simulink model "EnableBio1"  (R2017b)
settings: Solver=FixedStepDiscrete  StartTime=0.0  StopTime=10.0  FixedStep=0.200000  RelTol=1e-3  EnableMultiTasking=on
PreLoadFcn:
  | cellInfo = {
  |     { ...
  |          'cmp_cmd_msg' , ...
  |          '', ...
  |          sprintf(''), {  ...
  |                {  'apid', 1, 'uint16', -1, 'real', 'Sample' }; ...
  |                {  'sequence', 1, 'uint16', -1, 'real', 'Sample' }; ...
  |                {  'length', 1, 'uint16', -1, 'real', 'Sample' }; ...
  |                {  'command_id', 1, 'uint8', -1, 'real', 'Sample' }; ...
  |                {  'checksum', 1, 'uint8', -1, 'real', 'Sample' }; ...
  |                {  'params', 34, 'uint8', -1, 'real', 'Sample' }; ...
  |          }
  |     }
  | };
  | Simulink.Bus.cellToObject(cellInfo);
undefined symbols (not defined in the file): command_id, params, sequence
settings Model: Creator=hbourbou  LastModifiedBy=hbourbou
settings DataIOCC: LimitDataPoints=on
settings OptimizationCC: LifeSpan=inf
settings DebuggingCC: SFUnexpectedBacktrackingDiag=warning  SFNoUnconditionalDefaultTransitionDiag=warning  SFExecutionAtInitializationDiag=none
settings HardwareCC: ProdBitPerSizeT=32  ProdBitPerPtrDiffT=32  ProdWordSize=32  ProdHWDeviceType=Specified
settings ModelReferenceCC: PropagateSignalLabelsOutOfModel=off
settings CodeAppCC: StateflowObjectComments=on
settings GRTTargetCC: TargetLangStandard=C89/C90 (ANSI)
settings ConfigComp: CovMetricSettings=dw  CovHtmlReporting=on  CovSaveCumulativeToWorkspaceVar=on  CovSaveSingleToWorkspaceVar=on  CovExternalEMLEnable=off

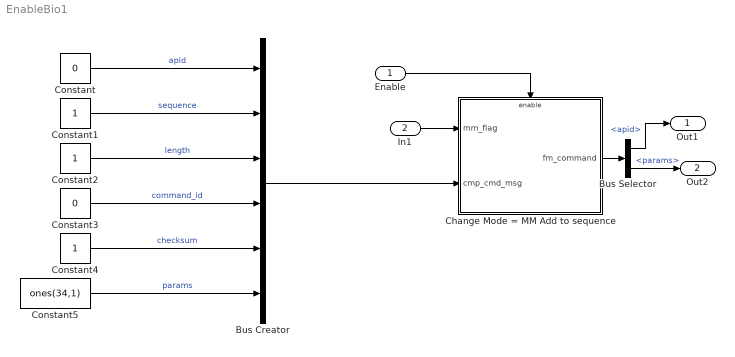
== system EnableBio1 ==
  Enable : Inport  OutDataTypeStr=boolean
  In1 : Inport  Port=2  OutDataTypeStr=uint8
  Bus Creator : BusCreator  Inputs=6  OutDataTypeStr=Bus: cmp_cmd_msg  NonVirtualBus=on
      settings: InheritFromInputs=off
  Bus Selector : BusSelector  OutputSignals=apid,params
  Change Mode = MM Add to sequence : Subsystem  TreatAsAtomicUnit=on
      settings: MinAlgLoopOccurrences=on
  Constant : Constant  Value=0  OutDataTypeStr=uint16
  Constant1 : Constant  OutDataTypeStr=uint16
  Constant2 : Constant  OutDataTypeStr=uint16
  Constant3 : Constant  Value=0  OutDataTypeStr=uint8
  Constant4 : Constant  OutDataTypeStr=uint8
  Constant5 : Constant  Value=ones(34,1)  OutDataTypeStr=uint8
  Out1 : Outport
  Out2 : Outport  Port=2
  wires:
  Change Mode = MM Add to sequence/1(fm_command) -> Bus Selector/1
  Enable/1 -> Change Mode = MM Add to sequence/Enable
  In1/1 -> Change Mode = MM Add to sequence/1(mm_flag)
  Constant4/1 -> Bus Creator/5  "checksum"
  Constant/1 -> Bus Creator/1  "apid"
  Constant5/1 -> Bus Creator/6  "params"
  Bus Creator/1 -> Change Mode = MM Add to sequence/2(cmp_cmd_msg)
  Constant1/1 -> Bus Creator/2  "sequence"
  Constant3/1 -> Bus Creator/4  "command_id"
  Constant2/1 -> Bus Creator/3  "length"
  Bus Selector/1 -> Out1/1  "<apid>"
  Bus Selector/2 -> Out2/1  "<params>"

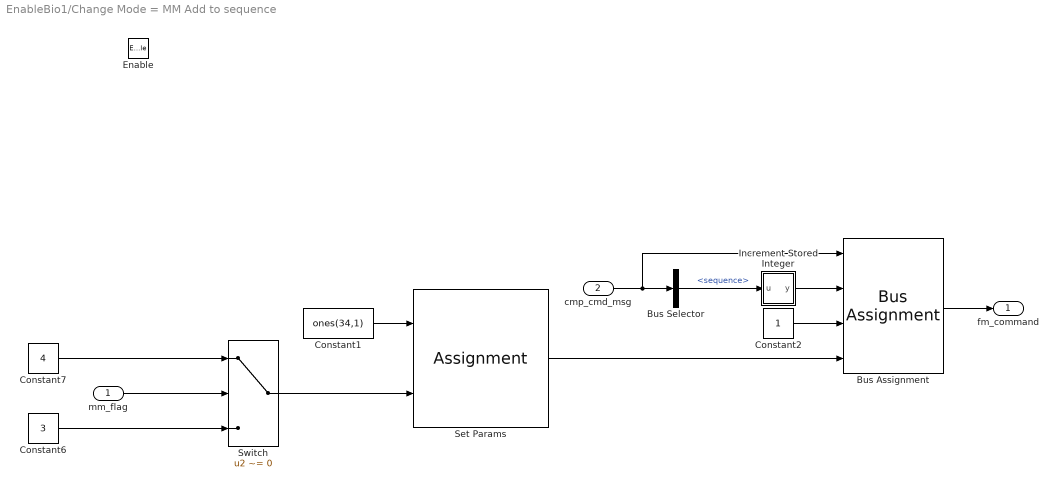
== system EnableBio1/Change Mode = MM Add to sequence ==
  mm_flag : Inport  OutDataTypeStr=uint8
  cmp_cmd_msg : Inport  Port=2  OutDataTypeStr=Bus: cmp_cmd_msg
  Enable : EnablePort
  Bus Assignment : BusAssignment  AssignedSignals=sequence,command_id,params
  Bus Selector : BusSelector  OutputSignals=sequence
  Constant1 : Constant  Value=ones(34,1)  OutDataTypeStr=uint8
  Constant2 : Constant  OutDataTypeStr=uint8
  Constant6 : Constant  Value=3  OutDataTypeStr=uint8
  Constant7 : Constant  Value=4  OutDataTypeStr=uint8
  Increment Stored Integer : Subsystem  AncestorBlock=|  TreatAsAtomicUnit=on  mask(Stored Integer Value Increment){}
      | simulink/Additional Math
      | & Discrete/Additional Math:
      | Increment - Decrement/Increment
      | Stored Integer
      mask help: Simulink:masks:StoredIntegerValueIncrement_MD
      settings: MinAlgLoopOccurrences=on
      mask Display: disp('Q++')
  Set Params : Assignment  DiagnosticForDimensions=Warning  IndexOptions=Index vector (dialog)  Indices=1  OutputSizes=1
  Switch : Switch  Criteria=u2 ~= 0
  fm_command : Outport
  wires:
  Constant2/1 -> Bus Assignment/3
  Bus Assignment/1 -> fm_command/1
  Increment Stored Integer/1(y) -> Bus Assignment/2
  Set Params/1 -> Bus Assignment/4
  Switch/1 -> Set Params/2
  Constant1/1 -> Set Params/1
  Bus Selector/1 -> Increment Stored Integer/1(u)  "<sequence>"
  cmp_cmd_msg/1 -> Bus Selector/1, Bus Assignment/1
  Constant7/1 -> Switch/1
  Constant6/1 -> Switch/3
  mm_flag/1 -> Switch/2

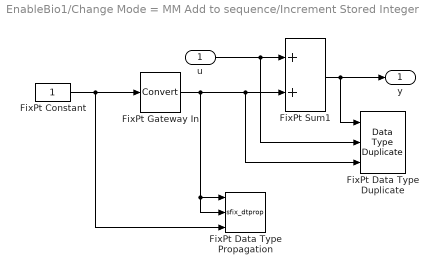
== system EnableBio1/Change Mode = MM Add to sequence/Increment Stored Integer ==
  u : Inport  OutDataTypeStr=uint16
  FixPt Constant : Constant  DisableCoverage=on  OutDataTypeStr=Inherit: Inherit via back propagation
  FixPt Data Type Duplicate : DataTypeDuplicate  DisableCoverage=on  NumInputPorts=3
  FixPt Data Type Propagation : S-Function  AncestorBlock=|  FunctionName=sfix_dtprop  Parameters=14,PropDataTypeMode,(getdatatypespecs(PropDataType,PropScaling,DblOver,0, 0, PropDataTypeMode, PropScalingMode)),IfRefDouble,IfRefSingle,IsSigned,NumBitsBase,NumBitsMult,NumBitsAdd,(sort(reshape(round(NumBitsAllowFinal), prod(size(NumBitsAllowFinal)),1))),PropScalingMode,ValuesUsedBestPrec,SlopeBase,SlopeMult,SlopeAdd,BiasBase,BiasMult,BiasAdd,DblOver  SFunctionDeploymentMode=off  EnableBusSupport=off  mask(Data Type Propagation){PropDataTypeMode=Inherit via propagation rule, PropDataType=fixdt(1, 16), IfRefDouble=double, IfRefSingle=single, IsSigned=IsSigned1, NumBitsBase=NumBits1, NumBitsMult=1, NumBitsAdd=0, NumBitsAllowFinal=1:128, PropScalingMode=Inherit via propagation rule, PropScaling=2^-10, ValuesUsedBestPrec=[5 -7], SlopeBase=Slope1, SlopeMult=0, SlopeAdd=1, BiasBase=Bias1, BiasMult=0, BiasAdd=0}
      | simulink/Signal
      | Attributes/Data Type
      | Propagation
      mask prompts: PropDataTypeMode "Simulink:masks:x1PropagatedDataType_MP"; PropDataType "Simulink:masks:x11PropagatedDataTypeegFixdt116Fixdtsingle_MP"; IfRefDouble "Simulink:masks:x11IfAnyReferenceInputIsDoubleOutputIs_MP"; IfRefSingle "Simulink:masks:x12IfAnyReferenceInputIsSingleOutputIs_MP"; IsSigned "Simulink:masks:x13IsSigned_MP"; NumBitsBase "Simulink:masks:x141NumberofBitsBase_MP"; NumBitsMult "Simulink:masks:x142NumberofBitsMultiplicativeAdjustment_MP"; NumBitsAdd "Simulink:masks:x143NumberofBitsAdditiveAdjustment_MP"; NumBitsAllowFinal "Simulink:masks:x144NumberofBitsAllowableFinalValues_MP"; PropScalingMode "Simulink:masks:x2PropagatedScaling_MP"; PropScaling "Simulink:masks:x21PropagatedScalingSlopeEg29OrSlopeBiasEg1253_MP"; ValuesUsedBestPrec "Simulink:masks:x21ValuesUsedToDetermineBestPrecisionScaling_MP"; SlopeBase "Simulink:masks:x211SlopeBase_MP"; SlopeMult "Simulink:masks:x212SlopeMultiplicativeAdjustment_MP"; SlopeAdd "Simulink:masks:x213SlopeAdditiveAdjustment_MP"; BiasBase "Simulink:masks:x221BiasBase_MP"; BiasMult "Simulink:masks:x222BiasMultiplicativeAdjustment_MP"; BiasAdd "Simulink:masks:x223BiasAdditiveAdjustment_MP"
      mask help: Simulink:masks:DataTypePropagation_MD
      mask init:
      | DblOver = 0;
      mask TypeOptions PropDataTypeMode: Simulink:masks:SpecifyViaDialog | Simulink:masks:InheritViaPropagationRule
      mask Callback PropDataTypeMode: fixptdialog(gcbh)
      mask Callback PropDataType: fixptdialog(gcbh)
      mask TypeOptions IfRefDouble: Simulink:masks:double | Simulink:masks:single
      mask TypeOptions IfRefSingle: Simulink:masks:double | Simulink:masks:single
      mask TypeOptions IsSigned: Simulink:masks:IsSigned1 | Simulink:masks:IsSigned2 | Simulink:masks:IsSigned1OrIsSigned2 | Simulink:masks:TRUE | Simulink:masks:FALSE
      mask TypeOptions NumBitsBase: NumBits1 | NumBits2 | max([NumBits1 NumBits2]) | min([NumBits1 NumBits2]) | NumBits1+NumBits2
      mask TypeOptions PropScalingMode: Simulink:masks:SpecifyViaDialog | Simulink:masks:InheritViaPropagationRule | Simulink:masks:ObtainViaBestPrecision
      mask Callback PropScalingMode: fixptdialog(gcbh)
      mask TypeOptions SlopeBase: Slope1 | Slope2 | max([Slope1 Slope2]) | min([Slope1 Slope2]) | Slope1*Slope2 | Slope1/Slope2 | PosRange1 | PosRange2 | max([PosRange1 PosRange2]) | min([PosRange1 PosRange2]) | PosRange1*PosRange2 | PosRange1/PosRange2
      mask TypeOptions BiasBase: Bias1 | Bias2 | max([Bias1 Bias2]) | min([Bias1 Bias2]) | Bias1*Bias2 | Bias1/Bias2 | Bias1+Bias2 | Bias1-Bias2
      mask Display:
      | port_label('Input',1,'Ref1');
      | port_label('Input',2,'Ref2');
      | port_label('Input',3,'Prop');
  FixPt Gateway In : DataTypeConversion  DisableCoverage=on  ConvertRealWorld=Stored Integer (SI)
  FixPt Sum1 : Sum  OutDataTypeStr=Inherit: Inherit via back propagation  InputSameDT=on  LockScale=on
  y : Outport
  wires:
  u/1 -> FixPt Data Type Duplicate/2, FixPt Sum1/1
  FixPt Constant/1 -> FixPt Gateway In/1, FixPt Data Type Propagation/3
  FixPt Sum1/1 -> FixPt Data Type Duplicate/1, y/1
  FixPt Gateway In/1 -> FixPt Data Type Duplicate/3, FixPt Sum1/2, FixPt Data Type Propagation/1, FixPt Data Type Propagation/2
